simulink model "pwm_model"  (R2024b)
settings: Solver=VariableStepAuto  StartTime=0.0  StopTime=0.2  RelTol=1e-3
libraries: spsPermanentMagnetSynchronousMachineLib x1, spsDCVoltageSourceLib x1, spsGroundLib x1, simulink x1, spsUniversalBridgeLib x1, sps_lib x1

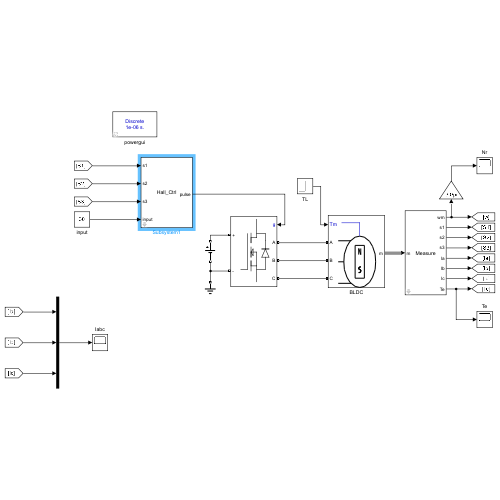
[thumbnail: Simulink's stored preview of the top-level diagram]
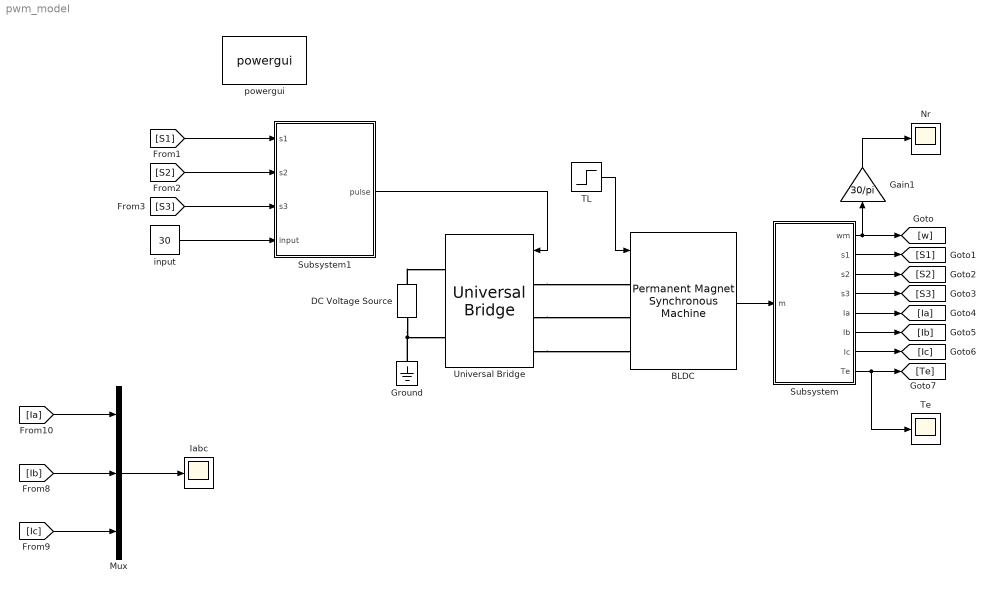
== system pwm_model ==
  BLDC : spsPermanentMagnetSynchronousMachineLib/Permanent Magnet Synchronous Machine  NbPhases=3  FluxDistribution=Trapezoidal  RotorType=Round  MechanicalLoad=Torque Tm  PresetModel=No  ShowDetailedParameters=on  MeasurementBus=off  Resistance=0.106/2  Inductance=0.000428/2  dqInductances=[8.5e-3,8.5e-3]  La=0.000395  MachineConstant=Torque Constant (N.m / A_peak)  Flux=0.041  VoltageCst=17.174  TorqueCst=0.164  Flat=120  Mechanical=[4943e-7 0.001 2 0]  PolePairs=4  InitialConditions=[0,0, 0,0]  InitialConditions5ph=[0 0 0 0 0 0]  RefAngle=Aligned with phase A axis (original Park)  IterativeDiscreteModel=Trapezoidal non iterative  TsBlock=-1  TsPowergui=0
  DC Voltage Source : spsDCVoltageSourceLib/DC Voltage Source  Amplitude=50  Measurements=None
  Gain1 : Gain  Gain=30/pi
  Ground : spsGroundLib/Ground  LConnTagsString=a
  Iabc : Scope
  Mux : Mux  Inputs=3
  Nr : Scope
  Subsystem : Subsystem
  Subsystem1 : Subsystem  mask{freq=10e3, Vdc=50}
      mask prompts: freq "freq : switch frequency"; Vdc "Vdc : bus voltage"
  TL : Step  Time=0.1  After=2  SampleTime=0
  Te : Scope
  Universal Bridge : spsUniversalBridgeLib/Universal Bridge  Arms=3  SnubberResistance=1e5  SnubberCapacitance=inf  Device=MOSFET / Diodes  Ron=1e-3  Lon=0  ForwardVoltages="[  0  0  ]"  ForwardVoltage=0  GTOparameters=[ 10e-6 , 20e-6 ]  IGBTparameters=[ 1e-6 , 2e-6 ]  Measurements=None  Measurements_2=None  converterType=Rectifier
  input : Constant  Value=30
  powergui : sps_lib/powergui  Priority=1  SimulationMode=Discrete  SampleTime=1e-6  frequency=60  Iterations=50  frequencyindice=0  Pbase=100e6  ErrMax=1e-4  UnitsV=kV  UnitsW=MW  buscounter=0  FunctionMessages=off  echomessages=off  EnableUseOfTLC=off  CurrentSourceSwitches=off  DisableSnubberDevices=off  DisableRonSwitches=off  DisableVfSwitches=off  DisplayEquations=off  AutomaticDiscreteSolvers=off  SolverType=Tustin/Backward Euler (TBE)  Interpol=off  ExternalGateDelay=off  methode=off  Ts=100  x0status=blocks  SPID=on  SwTol=0  HookPort=off  NonlinearTolerance=1e-4  nMaxIteration=100  ContinueOnMaxIteration=off  RestoreLinks=warning  ResistiveCurrentMeasurement=off  Frange=[0:2:500]  Ylog=off  Xlog=on  ShowGrid=off  save=off  variable=ZData  structure=0  ZoomFFT=off  StartTime=0.0  cycles=1  DisplayStyle=1  fundamental=60  FreqAxis=off  MaxFrequency=1000  frequencyindicesteady=1  RmsSteady=1  display=off
  wires:
  Mux/1 -> Iabc/1
  [Ic] -> Mux/3
  [Ia] -> Mux/1
  [Ib] -> Mux/2
  TL/1 -> BLDC/1
  BLDC/1 -> Subsystem/1(m)
  Subsystem/6(Ib) -> [Ib]
  Subsystem/2(s1) -> [S1]
  Subsystem/5(Ia) -> [Ia]
  Subsystem/7(Ic) -> [Ic]
  Subsystem/8(Te) -> Te/1, [Te]
  Subsystem/1(wm) -> Gain1/1, [w]
  Subsystem/3(s2) -> [S2]
  Gain1/1 -> Nr/1
  Subsystem/4(s3) -> [S3]
  [S1] -> Subsystem1/1(s1)
  [S2] -> Subsystem1/2(s2)
  [S3] -> Subsystem1/3(s3)
  input/1 -> Subsystem1/4(input)
  Subsystem1/1(pulse) -> Universal Bridge/1
  connections:
  Universal Bridge/LConn3 -- BLDC/LConn3
  Universal Bridge/LConn2 -- BLDC/LConn2
  Universal Bridge/LConn1 -- BLDC/LConn1
  DC Voltage Source/RConn1 -- Universal Bridge/RConn1
  DC Voltage Source/LConn1 -- Ground/LConn1 -- Universal Bridge/RConn2

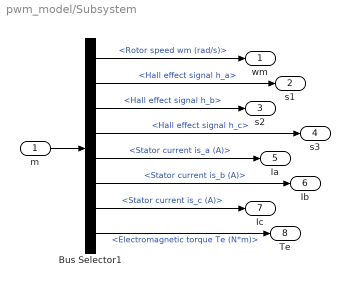
== system pwm_model/Subsystem ==
  m : Inport
  Bus Selector1 : BusSelector  OutputSignals=Rotor speed wm (rad/s),Hall effect signal h_a,Hall effect signal h_b,Hall effect signal h_c,Stator current is_a (A),Stator current is_b (A),Stator current is_c (A),Electromagnetic torque Te (N*m)
  wm : Outport
  s1 : Outport  Port=2
  s2 : Outport  Port=3
  s3 : Outport  Port=4
  Ia : Outport  Port=5
  Ib : Outport  Port=6
  Ic : Outport  Port=7
  Te : Outport  Port=8
  wires:
  m/1 -> Bus Selector1/1
  Bus Selector1/5 -> Ia/1  "<Stator current is_a (A)>"
  Bus Selector1/8 -> Te/1  "<Electromagnetic torque Te (N*m)>"
  Bus Selector1/6 -> Ib/1  "<Stator current is_b (A)>"
  Bus Selector1/7 -> Ic/1  "<Stator current is_c (A)>"
  Bus Selector1/1 -> wm/1  "<Rotor speed wm (rad/s)>"
  Bus Selector1/2 -> s1/1  "<Hall effect signal h_a>"
  Bus Selector1/3 -> s2/1  "<Hall effect signal h_b>"
  Bus Selector1/4 -> s3/1  "<Hall effect signal h_c>"

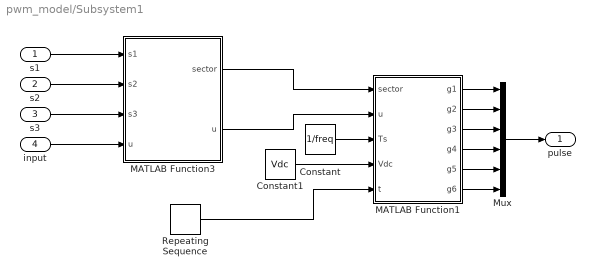
== system pwm_model/Subsystem1 ==
  s1 : Inport
  s2 : Inport  Port=2
  s3 : Inport  Port=3
  input : Inport  Port=4
  Constant : Constant  Value=1/freq
  Constant1 : Constant  Value=Vdc
  MATLAB Function1 : MATLAB Function  TreatAsAtomicUnit=on
  MATLAB Function3 : MATLAB Function  TreatAsAtomicUnit=on
  Mux : Mux  Inputs=6
  Repeating Sequence : simulink/Sources/Repeating Sequence  rep_seq_t=[0 1/(freq)]  rep_seq_y=[0 1/(freq)]
  pulse : Outport
  wires:
  s2/1 -> MATLAB Function3/2(s2)
  MATLAB Function3/2(u) -> MATLAB Function1/2(u)
  MATLAB Function3/1(sector) -> MATLAB Function1/1(sector)
  input/1 -> MATLAB Function3/4("u ")
  s1/1 -> MATLAB Function3/1(s1)
  s3/1 -> MATLAB Function3/3(s3)
  MATLAB Function1/1(g1) -> Mux/1
  MATLAB Function1/2(g2) -> Mux/2
  MATLAB Function1/3(g3) -> Mux/3
  MATLAB Function1/4(g4) -> Mux/4
  MATLAB Function1/5(g5) -> Mux/5
  MATLAB Function1/6(g6) -> Mux/6
  Mux/1 -> pulse/1
  Constant/1 -> MATLAB Function1/3(Ts)
  Constant1/1 -> MATLAB Function1/4(Vdc)
  Repeating Sequence/1 -> MATLAB Function1/5(t)

== matlab function pwm_model/Subsystem1/MATLAB Function3 ==
function [sector,u] = Hall_Table(s1,s2,s3,u)
    states = s1*4 + s2*2 + s3*1;
    if states == 0 || states == 7
        sector = 0;
        return;
    end
    %map table
    map_tab = [6, 4, 5, 2, 1, 3];
    if u > 0 
        dir = 1;
    else
        dir = -1;
        u = -u;
    end

    if dir > 0 %CCW, forward rotation
        sector = map_tab(states);
    else %CW, reversal rotation
        sector = mod(map_tab(states) - 1 + 3,6) + 1;
    end
end

== matlab function pwm_model/Subsystem1/MATLAB Function1 ==
function [g1,g2,g3,g4,g5,g6] = my_PWM(sector,u,Ts,Vdc,t)
   if u >= Vdc  %u >= 0
       u = Vdc;
   end

   t1 = [u/Vdc*Ts,Ts];%use this method to simulate PWM pulse output
   g_num = [1 0];
   for j = 1:2
       if t < t1(j)
           break;
       end
   end
   g = g_num(j);
   switch sector
       case 1
           pulses = [g,0,0,1,0,0];
       case 2
           pulses = [g,0,0,0,0,1];
       case 3
           pulses = [0,0,g,0,0,1];
       case 4
           pulses = [0,1,g,0,0,0];
       case 5
           pulses = [0,1,0,0,g,0];
       case 6
           pulses = [0,0,0,1,g,0];
       otherwise
           pulses = [0,0,0,0,0,0];
   end
g1 = pulses(1);
g2 = pulses(2);
g3 = pulses(3);
g4 = pulses(4);
g5 = pulses(5);
g6 = pulses(6);
